simulink model "SubSnapSlow"  (R2020a)
settings: configuration reference "cigreConfig" (kept outside this file)
model workspace (MAT data in the model file):
  sub_param = Simulink.Parameter
  sub_param.Value = 6
  sub_param.DataType = 'int32'
  sub_param.Complexity = 'real'
  sub_param.Dimensions = [1 1]
settings Model: DataDictionary=MySLDD.sldd  OrderedModelArguments=off  Creator=raarenst  LastModifiedBy=toma
settings ConfigSetRef: SourceName=cigreConfig

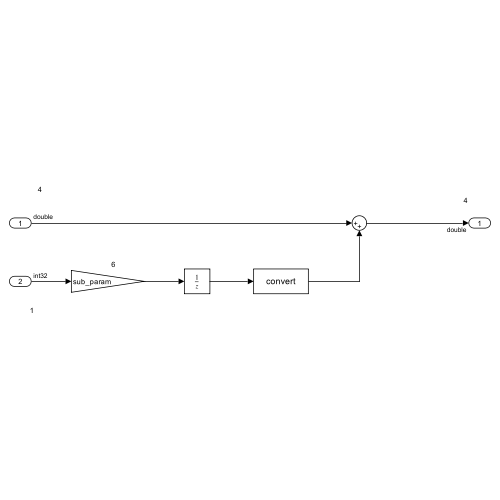
[thumbnail: Simulink's stored preview of the top-level diagram]
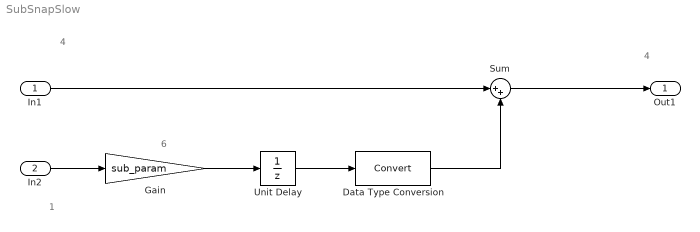
== system SubSnapSlow ==
  note: 6
  note: 4
  note: 4
  note: 1
  In1 : Inport  OutDataTypeStr=double  SampleTime=1
  In2 : Inport  Port=2  OutDataTypeStr=int32  SampleTime=1
  Data Type Conversion : DataTypeConversion
  Gain : Gain  Gain=sub_param  ParamDataTypeStr=int32  OutDataTypeStr=int32
  Sum : Sum  Inputs=|++
  Unit Delay : UnitDelay  SampleTime=-1  HasFrameUpgradeWarning=on
  Out1 : Outport  OutDataTypeStr=double
  wires:
  In2/1 -> Gain/1
  Gain/1 -> Unit Delay/1
  Unit Delay/1 -> Data Type Conversion/1
  In1/1 -> Sum/1
  Data Type Conversion/1 -> Sum/2
  Sum/1 -> Out1/1
